simulink model "CarE_Model"  (R2019b)
settings: Solver=VariableStepAuto  StartTime=0.0  StopTime=inf  RelTol=1e-3
(part 1 of 5)
settings Model: EnablePacing=on  Creator=20175127  LastModifiedBy=XPS13
settings DataIOCC: ReturnWorkspaceOutputs=off
settings DebuggingCC: ArithmeticOperatorsInVariantConditions=warning
settings SFSimCC: CustomCodeUndefinedFunction=UseInterfaceOnly

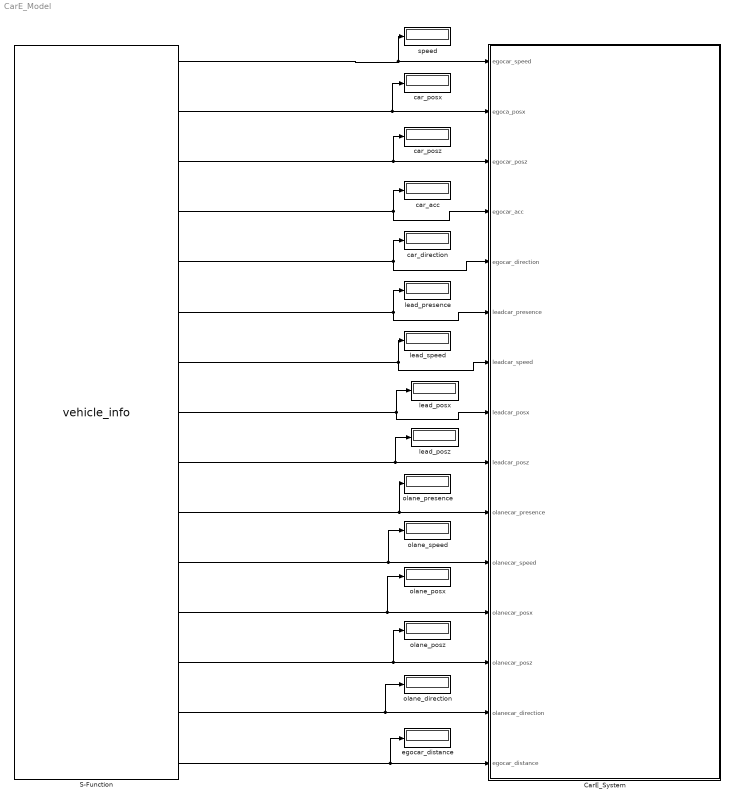
== system CarE_Model ==
  CarE_System : Subsystem
  S-Function : S-Function  FunctionName=vehicle_info  SFunctionDeploymentMode=off  EnableBusSupport=off
  car_acc : Display
  car_direction : Display
  car_posx : Display
  car_posz : Display
  egocar_distance : Display
  lead_posx : Display
  lead_posz : Display
  lead_presence : Display
  lead_speed : Display
      settings: Decimation=5
  olane_direction : Display
  olane_posx : Display
  olane_posz : Display
  olane_presence : Display
  olane_speed : Display
      settings: Decimation=5
  speed : Display
      settings: Decimation=5
  wires:
  S-Function/1 -> CarE_System/1(egocar_speed), speed/1
  S-Function/2 -> car_posx/1, CarE_System/2(egoca_posx)
  S-Function/3 -> CarE_System/3(egocar_posz), car_posz/1
  S-Function/4 -> CarE_System/4(egocar_acc), car_acc/1
  S-Function/5 -> CarE_System/5(egocar_direction), car_direction/1
  S-Function/6 -> CarE_System/6(leadcar_presence), lead_presence/1
  S-Function/7 -> lead_speed/1, CarE_System/7(leadcar_speed)
  S-Function/8 -> CarE_System/8(leadcar_posx), lead_posx/1
  S-Function/9 -> CarE_System/9(leadcar_posz), lead_posz/1
  S-Function/10 -> olane_presence/1, CarE_System/10(olanecar_presence)
  S-Function/11 -> CarE_System/11(olanecar_speed), olane_speed/1
  S-Function/12 -> CarE_System/12(olanecar_posx), olane_posx/1
  S-Function/13 -> olane_posz/1, CarE_System/13(olanecar_posz)
  S-Function/14 -> olane_direction/1, CarE_System/14(olanecar_direction)
  S-Function/15 -> CarE_System/15(egocar_distance), egocar_distance/1

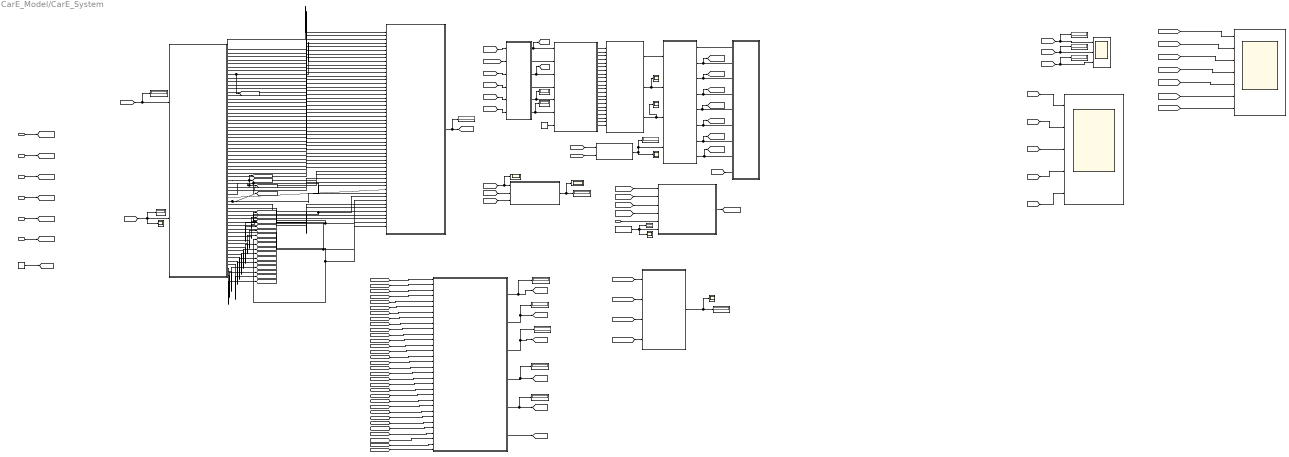
== system CarE_Model/CarE_System ==
  note: Input from unity
  note: output from simulink
  egocar_speed : Inport
  egoca_posx : Inport  Port=2
  egocar_posz : Inport  Port=3
  egocar_acc : Inport  Port=4
  egocar_direction : Inport  Port=5
  leadcar_presence : Inport  Port=6
  leadcar_speed : Inport  Port=7
  leadcar_posx : Inport  Port=8
  leadcar_posz : Inport  Port=9
  olanecar_presence : Inport  Port=10
  olanecar_speed : Inport  Port=11
  olanecar_posx : Inport  Port=12
  olanecar_posz : Inport  Port=13
  olanecar_direction : Inport  Port=14
  egocar_distance : Inport  Port=15
  Display{5..9,11..13} (8 alike) : Display
  Emotion Module : Subsystem
  Emotion_Intensity_Input_Module : Subsystem
  Event_detect_module : Subsystem
  Events-Agent-Event-Action : Scope  NumInputPorts=3
  HF : Display
  HF_normal : Display
  Health_Module_2.0 : Subsystem
  Input_module_2.0 : Subsystem
  MATLAB Function : MATLAB Function  TreatAsAtomicUnit=on
  Mapping Module : Subsystem
  Mood Module : Subsystem
  Optimization_module : Subsystem
  Output Module : Subsystem
  Personality_module : Subsystem
  S-Function1 : S-Function  FunctionName=curve_event  SFunctionDeploymentMode=off  EnableBusSupport=off
  Scope{,1..5} (6 alike) : Scope
  Sress factors : Scope  NumInputPorts=5
  Stress_module : Subsystem
  average_speed_data_mps : Constant  Value=14.72
  basic_emotions : Scope  NumInputPorts=7
  curve_trigger : Display
  fix_LoS : Constant
  gap : Scope
  sf_Env : Display
  sf_VC : Display
  sf_VH : Display
  sf_driving : Display
  sf_total : Display
  speed _CAR : Scope
  utility : Display
  wires:
  Input_module_2.0/16(axle_st) -> Health_Module_2.0/16(axle_st)
  Input_module_2.0/43(bigdata_connection_st) -> Health_Module_2.0/43(bigdata_connection_st), [bigdata_st]
  Input_module_2.0/8(maintanance_periodicity_st) -> Health_Module_2.0/8(maintenance_periodicity_st)
  Input_module_2.0/2(driver_alcohol_st) -> Health_Module_2.0/2(driver_alcohol_st)
  Input_module_2.0/13(service_brak_st) -> Health_Module_2.0/13(serv_brake_PE_st)
  Input_module_2.0/31(telltales_st) -> Health_Module_2.0/31(telltales_st)
  Input_module_2.0/33(wheel_st) -> Health_Module_2.0/33(wheel_st)
  Input_module_2.0/42(software_freq_st) -> Health_Module_2.0/42(software_freq_st)
  Input_module_2.0/51(cab_humiity_st) -> Health_Module_2.0/51(cab_humidity_st)
  Input_module_2.0/14(second_brake_st) -> Health_Module_2.0/14(second_brake_st)
  Input_module_2.0/21(reverse_lamps_st) -> Health_Module_2.0/21(reverse_lamp_st)
  Input_module_2.0/36(chassis_st) -> Health_Module_2.0/36(chassis_st)
  Input_module_2.0/25(steering_st) -> Health_Module_2.0/25(steering_st)
  Input_module_2.0/38(obt_recog_st) -> Health_Module_2.0/38(obt_recog_st)
  Input_module_2.0/32(wheelhub_st) -> Health_Module_2.0/32(wheel_hub_st)
  Input_module_2.0/9(gap_st) -> Health_Module_2.0/9(grap_st), [gap_st]
  Input_module_2.0/24(seat_st) -> Health_Module_2.0/24(seat_st)
  Input_module_2.0/5(driver_workload_st) -> Health_Module_2.0/5(driver_workload_st)
  Input_module_2.0/23(airbag_st) -> Health_Module_2.0/23(airbag_st)
  Input_module_2.0/3(driver_alertness_st) -> Health_Module_2.0/3(driver_alertness_st)
  Input_module_2.0/1(driver_age_st) -> Health_Module_2.0/1(driver_age_st)
  Input_module_2.0/18(door_st) -> Health_Module_2.0/18(door_st)
  Input_module_2.0/41(Friendly_HM_interaction_st) -> Health_Module_2.0/41(friendly_HM_interaction_st)
  Input_module_2.0/4(driver_vision_st) -> Health_Module_2.0/4(driver_vision_st)
  Input_module_2.0/11(vehicle_mass_st) -> Health_Module_2.0/11(vehicle_mass_st)
  Input_module_2.0/39(v2v_st) -> Health_Module_2.0/39(v2v_st), [v2v_st]
  Input_module_2.0/53(weather_st) -> Health_Module_2.0/53(weather_st), [weather_st]
  Input_module_2.0/46(road_surface_st) -> [road_surface_st], Health_Module_2.0/46(road_surface_st)
  Input_module_2.0/48(prob_acc_road_st) -> Health_Module_2.0/48(prob_acc_road_st)
  Input_module_2.0/27(eps_st) -> Health_Module_2.0/27(eps_st)
  Input_module_2.0/49(prob_construction_st) -> Health_Module_2.0/49(prob_construction_st)
  Input_module_2.0/54(time_of_day_st) -> [time_of_day_st], Health_Module_2.0/54(time_of_day_st)
  Input_module_2.0/20(head_lamp_st) -> Health_Module_2.0/20(headlamp_st)
  Input_module_2.0/47(road_condition_st) -> [road_condition_st], Health_Module_2.0/47(road_condition_st)
  Input_module_2.0/40(v2i_st) -> Health_Module_2.0/40(v2i_st), [v2i_st]
  Input_module_2.0/6(driver_emotion_st) -> Health_Module_2.0/6(driver_emotion_st)
  Input_module_2.0/12(brakes_st) -> Health_Module_2.0/12(brakes_st)
  Input_module_2.0/10("speeding_freq_st ") -> Health_Module_2.0/10(speeding_freq_st)
  Input_module_2.0/45(cooperative_driving_st) -> Health_Module_2.0/45(cooperative_driving_st), [cooperative_dr_st]
  Input_module_2.0/7(driver_attitude_st) -> Health_Module_2.0/7(driver_attitude_st)
  Input_module_2.0/19(fog_lamp_st) -> Health_Module_2.0/19(fog_lamp_st)
  Input_module_2.0/44(digital_user_interface_st) -> Health_Module_2.0/44(digital_user_interface_st)
  Input_module_2.0/52(driving_env_contition) -> Health_Module_2.0/52(driving_env_condition_st)
  Input_module_2.0/26(wheel_alignment_st) -> Health_Module_2.0/26(wheel_alignment_st)
  Input_module_2.0/50(cab_temperature_st) -> Health_Module_2.0/50(cab_temperature_st)
  Input_module_2.0/22(belts_st) -> Health_Module_2.0/22(belts_st)
  Input_module_2.0/15(parking_brake_st) -> Health_Module_2.0/15(parkin_brake_st)
  Input_module_2.0/28(streering_wheel_st) -> Health_Module_2.0/28(steering_wheel_st)
  Input_module_2.0/29(stop_lamp_st) -> Health_Module_2.0/29(stop_lamps_st)
  Input_module_2.0/30(suspension_st) -> Health_Module_2.0/30(suspension_st)
  Input_module_2.0/37(noise_st) -> Health_Module_2.0/37(noise_st)
  Input_module_2.0/35(cabine_st) -> Health_Module_2.0/35(cabine_st)
  Input_module_2.0/34(tyre_st) -> Health_Module_2.0/34(tyre_st)
  Input_module_2.0/17(warm_lamp_st) -> Health_Module_2.0/17(warm_lamp_st)
  Emotion Module/21(liking_dec) -> Mood Module/21(liking_dec)
  Emotion Module/8(disappointment_dec) -> Mood Module/8(disappointment_dec)
  Emotion Module/15(admiration_dec) -> Mood Module/15(admiration_dec)
  Mapping Module/8(surprise_val) -> [surprise_val], Output Module/8(surprise_val)
  Mapping Module/5(happiness_val) -> Output Module/5(happiness_val), [happiness_val]
  Emotion Module/11(gloating_dec) -> Mood Module/11(gloating_dec)
  Emotion Module/4(fear_dec) -> Mood Module/4(fear_dec)
  Mapping Module/7(sadness_val) -> Output Module/7(sadness_val), [sadness_val]
  Emotion Module/12(resentment_dec) -> Mood Module/12(resentment_dec)
  Emotion Module/6(fear_confirmed_dec) -> Mood Module/6(fear_confirmed_dec)
  Emotion Module/14(shame_dec) -> Mood Module/14(shame_dec)
  Mapping Module/1(mood_val) -> Output Module/1(mood)
  Mapping Module/6(neutral_val) -> Output Module/6(neutral_val), [neutral_val]
  Mood Module/1(mood) -> Mapping Module/1(mood)
  Emotion Module/20(remorse_dec) -> Mood Module/20(remorse_dec)
  Emotion Module/3(hope_dec) -> Mood Module/3(hope_dec)
  Mood Module/2(contribution) -> Scope1/1, Mapping Module/2(contribution)
  Mood Module/3(index) -> Scope/1, Mapping Module/3(index)
  Emotion Module/7(relief_dec) -> Mood Module/7(relief_dec)
  Emotion Module/18(anger_dec) -> Mood Module/18(anger_dec)
  Emotion Module/19(gratification_dec) -> Mood Module/19(gratification_dec)
  Emotion Module/1(joy_dec) -> Mood Module/1(joy_dec)
  Mapping Module/3(disgust_val) -> Output Module/3(disgust_val), [disgust_val]
  Emotion Module/9(happy_for_dec) -> Mood Module/9(happy_for_dec)
  Emotion Module/5(satisfaction_dec) -> Mood Module/5(satisfaction_dec)
  Emotion Module/2("distress_dec ") -> Mood Module/2(distress_dec)
  Emotion Module/16(reproach_dec) -> Mood Module/16(reproach_dec)
  Emotion Module/13(pride_dec) -> Mood Module/13(pride_dec)
  Mapping Module/2(anger_val) -> [anger_val], Output Module/2(anger_val)
  Mapping Module/4(fear_val) -> [fear_val], Output Module/4(fear_val)
  Emotion Module/22(disliking_dec) -> Mood Module/22(disliking_dec)
  Emotion Module/10(sorry_for_dec) -> Mood Module/10(sorry_for_dec)
  Emotion Module/17(gratitude_dec) -> Mood Module/17(gratitude_dec)
  leadcar_presence/1 -> Event_detect_module/5(leadcar_presence)
  olanecar_presence/1 -> [olanecar_presence]
  S-Function1/1 -> Event_detect_module/6(curve_trigger), curve_trigger/1, Scope4/1
  Health_Module_2.0/1(Health_Factor) -> HF_normal/1, [health_factor]
  egoca_posx/1 -> [egocar_posx]
  egocar_posz/1 -> [egocar_posz]
  egocar_direction/1 -> [egocar_direction]
  egocar_speed/1 -> [egocar_speed]
  Input_module_2.0/55(r_personality) -> [r_personality]
  olanecar_speed/1 -> Stress_module/28(olanecar_speed)
  olanecar_posx/1 -> Stress_module/25(olanecar_posx)
  olanecar_posz/1 -> Stress_module/26(olanecar_posz)
  olanecar_direction/1 -> Stress_module/27(olanecar_direction)
  leadcar_posz/1 -> Stress_module/22(leadcar_posz)
  leadcar_posx/1 -> Stress_module/21(leadcar_posx)
  leadcar_speed/1 -> Stress_module/23(leadcar_speed)
  egocar_acc/1 -> Stress_module/15(egocar_acceleration)
  Event_detect_module/1(event_id) -> [scenario_id]
  Input_module_2.0/56(avg_accident_road) -> [avg_acc_road]
  Input_module_2.0/57(sd_accident_road) -> [sd_acc_road]
  Input_module_2.0/58(accidents_road) -> [acc_road]
  Input_module_2.0/60(Un_Obj_recog) -> [uncertainty_obj_recog]
  Input_module_2.0/59(avg_gap) -> [avg_gap]
  Personality_module/1(Utility) -> Scope2/1, utility/1
  Stress_module/2(Sf_Env) -> [sf_env], sf_Env/1
  Stress_module/1(Sf_VH) -> [sf_vh], sf_VH/1
  Stress_module/5(Sf_driving) -> sf_driving/1, [sf_driving]
  Stress_module/4(sf_VC) -> [sf_vc], sf_VC/1
  Input_module_2.0/64(pedestrian_active) -> [pedestrian_active]
  Input_module_2.0/65(legal_speed) -> [legal_speed]
  Emotion_Intensity_Input_Module/5(LoS) -> Display5/1, Emotion Module/5(LoS)
  Emotion_Intensity_Input_Module/6(LoF) -> Display6/1, Emotion Module/6(LoF)
  Emotion_Intensity_Input_Module/4(action_id) -> Emotion Module/4(action_id)
  Emotion_Intensity_Input_Module/3(event_id) -> [event_id], Emotion Module/3(event_id)
  Emotion_Intensity_Input_Module/2(agent_id) -> Emotion Module/2(agent_id)
  Input_module_2.0/61(rate_acceleration) -> [rate_acceleration]
  Input_module_2.0/62(rate_desceleration) -> [rate_desceleration]
  Input_module_2.0/63(average_speed) -> [avg_speed]
  Stress_module/3(SF_total) -> [stress_factor], sf_total/1
  Input_module_2.0/66(max_car_speed) -> [max_car_speed]
  egocar_distance/1 -> [ego_distance]
  fix_LoS/1 -> Emotion Module/7(fix_loS)
  average_speed_data_mps/1 -> [av_speed_data]
  Optimization_module/1(suggested_speed) -> Scope3/1, Display9/1
  MATLAB Function/1(HF_modified) -> Scope5/1, HF/1, Mapping Module/4(health_factor)
  [ego_distance] -> Input_module_2.0/1(distance), Display8/1
  [ego_distance] -> Stress_module/1(egocar_distance)
  [olanecar_presence] -> Event_detect_module/4(olanecar_presence)
  [olanecar_presence] -> Stress_module/24(olanecar_prescence)
  [egocar_speed] -> speed _CAR/1, Personality_module/1(egocar_speed)
  [egocar_speed] -> Stress_module/9(egocar_speed)
  [egocar_speed] -> Emotion_Intensity_Input_Module/5(egocar_speed)
  [r_personality] -> Personality_module/3(r_personality)
  [max_car_speed] -> Personality_module/2(egocar_max_speed)
  [egocar_posx] -> Event_detect_module/1(egocar_posx)
  [egocar_posx] -> Stress_module/18(egocar_posx)
  [egocar_posz] -> Stress_module/19(egocar_posz)
  [egocar_direction] -> Stress_module/20(egocar_direction)
  [egocar_posz] -> Event_detect_module/2(egocar_posz)
  [egocar_direction] -> Event_detect_module/3(egocar_direction)
  [scenario_id] -> Stress_module/16(event_id)
  [scenario_id] -> Optimization_module/3(event_ID)
  [scenario_id] -> Emotion_Intensity_Input_Module/1(event_ID)
  [scenario_id] -> Events-Agent-Event-Action/1, Display7/1
  Stress_module/6(gap) -> [gap]
  [gap] -> Display11/1, gap/1, Input_module_2.0/2(gap)
  [health_factor] -> MATLAB Function/1(Health_factor)
  [stress_factor] -> Output Module/9(stress_val)
  [stress_factor] -> MATLAB Function/2(SF)
  [stress_factor] -> Emotion_Intensity_Input_Module/3(sf_total)
  [stress_factor] -> Sress factors/5
  [sf_vc] -> Sress factors/3
  [sf_driving] -> Sress factors/4
  [sf_vc] -> Optimization_module/2(SF_VC)
  [sf_vh] -> Optimization_module/1(SF_VH)
  [sf_env] -> Sress factors/2
  [sf_vh] -> Sress factors/1
  [av_speed_data] -> Stress_module/32(avg_speed_data)
  [av_speed_data] -> Optimization_module/4(avgspeed_data)
  [avg_acc_road] -> Stress_module/2(avg_accidents_road)
  [sd_acc_road] -> Stress_module/3(sd_accidents_road)
  [acc_road] -> Stress_module/4(accidents_road)
  [avg_gap] -> Stress_module/17(avg_gap)
  [uncertainty_obj_recog] -> Stress_module/10(un_obj_recog)
  [rate_acceleration] -> Stress_module/30(rate_acceleration)
  [rate_desceleration] -> Stress_module/31(rate_desceleration)
  [avg_speed] -> Stress_module/29(average_speed)
  [pedestrian_active] -> Emotion_Intensity_Input_Module/2(event_0)
  [legal_speed] -> Emotion_Intensity_Input_Module/6(maxlegal_speed)
  [gap_st] -> Emotion_Intensity_Input_Module/4(gap_st)
  [goal_ID] -> Display12/1, Events-Agent-Event-Action/2
  [event_id] -> Events-Agent-Event-Action/3, Display13/1
  Emotion_Intensity_Input_Module/1(goal_id) -> [goal_ID], Emotion Module/1(goal_id)
  [v2v_st] -> Stress_module/11(v2v_st)
  [v2i_st] -> Stress_module/12(v2i_st)
  [bigdata_st] -> Stress_module/13(bigdata_connection_st)
  [cooperative_dr_st] -> Stress_module/14(cooperative_driving_st)
  [road_surface_st] -> Stress_module/5(road_surface_st)
  [road_condition_st] -> Stress_module/6(road_condition_st)
  [weather_st] -> Stress_module/7(weather_condition_st)
  [time_of_day_st] -> Stress_module/8(time_day_st)
  [anger_val] -> basic_emotions/1
  [disgust_val] -> basic_emotions/2
  [fear_val] -> basic_emotions/3
  [happiness_val] -> basic_emotions/4
  [neutral_val] -> basic_emotions/5
  [sadness_val] -> basic_emotions/6
  [surprise_val] -> basic_emotions/7

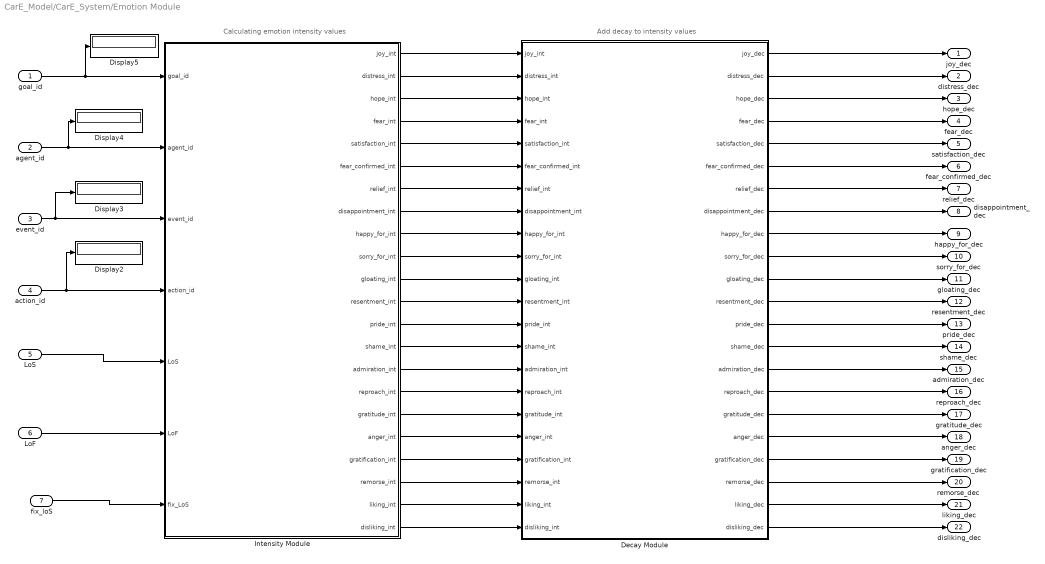
== system CarE_Model/CarE_System/Emotion Module ==
  note: Calculating emotion intensity values
  note: Add decay to intensity values
  goal_id : Inport
  agent_id : Inport  Port=2
  event_id : Inport  Port=3
  action_id : Inport  Port=4
  LoS : Inport  Port=5
  LoF : Inport  Port=6
  fix_loS : Inport  Port=7
  Decay Module : Subsystem
  Display{2..5} (4 alike) : Display
  Intensity Module : Subsystem
  joy_dec : Outport  VectorParamsAs1DForOutWhenUnconnected=off
  "distress_dec " : Outport  Port=2  VectorParamsAs1DForOutWhenUnconnected=off
  hope_dec : Outport  Port=3  VectorParamsAs1DForOutWhenUnconnected=off
  fear_dec : Outport  Port=4  VectorParamsAs1DForOutWhenUnconnected=off
  satisfaction_dec : Outport  Port=5  VectorParamsAs1DForOutWhenUnconnected=off
  fear_confirmed_dec : Outport  Port=6  VectorParamsAs1DForOutWhenUnconnected=off
  relief_dec : Outport  Port=7  VectorParamsAs1DForOutWhenUnconnected=off
  disappointment_dec : Outport  Port=8  VectorParamsAs1DForOutWhenUnconnected=off
  happy_for_dec : Outport  Port=9  VectorParamsAs1DForOutWhenUnconnected=off
  sorry_for_dec : Outport  Port=10  VectorParamsAs1DForOutWhenUnconnected=off
  gloating_dec : Outport  Port=11  VectorParamsAs1DForOutWhenUnconnected=off
  resentment_dec : Outport  Port=12  VectorParamsAs1DForOutWhenUnconnected=off
  pride_dec : Outport  Port=13  VectorParamsAs1DForOutWhenUnconnected=off
  shame_dec : Outport  Port=14  VectorParamsAs1DForOutWhenUnconnected=off
  admiration_dec : Outport  Port=15  VectorParamsAs1DForOutWhenUnconnected=off
  reproach_dec : Outport  Port=16  VectorParamsAs1DForOutWhenUnconnected=off
  gratitude_dec : Outport  Port=17  VectorParamsAs1DForOutWhenUnconnected=off
  anger_dec : Outport  Port=18  VectorParamsAs1DForOutWhenUnconnected=off
  gratification_dec : Outport  Port=19  VectorParamsAs1DForOutWhenUnconnected=off
  remorse_dec : Outport  Port=20  VectorParamsAs1DForOutWhenUnconnected=off
  liking_dec : Outport  Port=21  VectorParamsAs1DForOutWhenUnconnected=off
  disliking_dec : Outport  Port=22  VectorParamsAs1DForOutWhenUnconnected=off
  wires:
  goal_id/1 -> Display5/1, Intensity Module/1(goal_id)
  agent_id/1 -> Intensity Module/2(agent_id), Display4/1
  Intensity Module/1(joy_int) -> Decay Module/1(joy_int)
  Intensity Module/2("distress_int ") -> Decay Module/2(distress_int)
  Intensity Module/3(hope_int) -> Decay Module/3(hope_int)
  Intensity Module/4(fear_int) -> Decay Module/4(fear_int)
  Intensity Module/5(satisfaction_int) -> Decay Module/5(satisfaction_int)
  Intensity Module/6(fear_confirmed_int) -> Decay Module/6(fear_confirmed_int)
  Intensity Module/7(relief_int) -> Decay Module/7(relief_int)
  Intensity Module/8(disappointment_int) -> Decay Module/8(disappointment_int)
  Intensity Module/9(happy_for_int) -> Decay Module/9(happy_for_int)
  Intensity Module/10(sorry_for_int) -> Decay Module/10(sorry_for_int)
  Intensity Module/11(gloating_int) -> Decay Module/11(gloating_int)
  Intensity Module/12(resentment_int) -> Decay Module/12(resentment_int)
  Intensity Module/13(pride_int) -> Decay Module/13(pride_int)
  Intensity Module/14(shame_int) -> Decay Module/14(shame_int)
  Intensity Module/15(admiration_int) -> Decay Module/15(admiration_int)
  Intensity Module/16(reproach_int) -> Decay Module/16(reproach_int)
  Intensity Module/17(gratitude_int) -> Decay Module/17(gratitude_int)
  Intensity Module/18(anger_int) -> Decay Module/18(anger_int)
  Intensity Module/19(gratification_int) -> Decay Module/19(gratification_int)
  Intensity Module/20(remorse_int) -> Decay Module/20(remorse_int)
  Intensity Module/21(liking_int) -> Decay Module/21(liking_int)
  Intensity Module/22(disliking_int) -> Decay Module/22(disliking_int)
  Decay Module/10(sorry_for_dec) -> sorry_for_dec/1
  Decay Module/5(satisfaction_dec) -> satisfaction_dec/1
  Decay Module/11(gloating_dec) -> gloating_dec/1
  Decay Module/7(relief_dec) -> relief_dec/1
  Decay Module/16(reproach_dec) -> reproach_dec/1
  Decay Module/21(liking_dec) -> liking_dec/1
  Decay Module/14(shame_dec) -> shame_dec/1
  Decay Module/13(pride_dec) -> pride_dec/1
  Decay Module/1(joy_dec) -> joy_dec/1
  Decay Module/3(hope_dec) -> hope_dec/1
  Decay Module/17(gratitude_dec) -> gratitude_dec/1
  Decay Module/9(happy_for_dec) -> happy_for_dec/1
  Decay Module/20(remorse_dec) -> remorse_dec/1
  Decay Module/19(gratification_dec) -> gratification_dec/1
  Decay Module/2("distress_dec ") -> "distress_dec "/1
  Decay Module/22(disliking_dec) -> disliking_dec/1
  Decay Module/18(anger_dec) -> anger_dec/1
  Decay Module/6(fear_confirmed_dec) -> fear_confirmed_dec/1
  Decay Module/8(disappointment_dec) -> disappointment_dec/1
  Decay Module/15(admiration_dec) -> admiration_dec/1
  Decay Module/12(resentment_dec) -> resentment_dec/1
  Decay Module/4(fear_dec) -> fear_dec/1
  event_id/1 -> Intensity Module/3(event_id), Display3/1
  action_id/1 -> Intensity Module/4(action_id), Display2/1
  fix_loS/1 -> Intensity Module/7(fix_LoS)
  LoF/1 -> Intensity Module/6(LoF)
  LoS/1 -> Intensity Module/5(LoS)

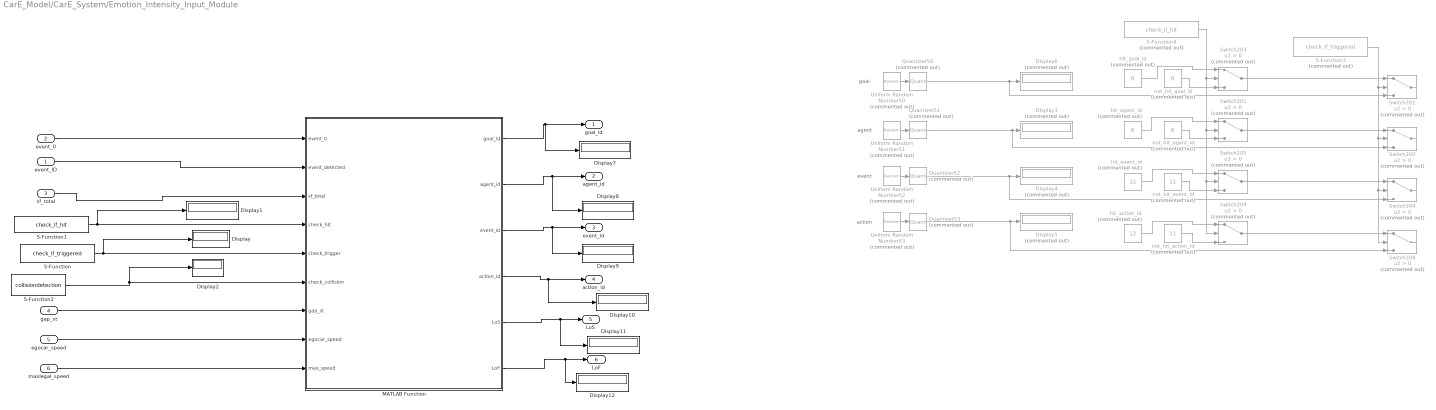
== system CarE_Model/CarE_System/Emotion_Intensity_Input_Module ==
  note: goal
  note: agent
  note: event
  note: action
  event_ID : Inport
  event_0 : Inport  Port=2
  sf_total : Inport  Port=3
  gap_st : Inport  Port=4
  egocar_speed : Inport  Port=5
  maxlegal_speed : Inport  Port=6
  Display{,1..2,7..12} (9 alike) : Display
  Display{3..6} (4 alike) : Display  Commented=on
  MATLAB Function : MATLAB Function  TreatAsAtomicUnit=on
  Quantizer{50..53} (4 alike) : Quantizer  Commented=on  QuantizationInterval=1
  S-Function : S-Function  FunctionName=check_if_triggered  SFunctionDeploymentMode=off  EnableBusSupport=off
  S-Function1 : S-Function  FunctionName=check_if_hit  SFunctionDeploymentMode=off  EnableBusSupport=off
  S-Function2 : S-Function  FunctionName=collisiondetection  SFunctionDeploymentMode=off  EnableBusSupport=off
  S-Function3 : S-Function  Commented=on  FunctionName=check_if_triggered  SFunctionDeploymentMode=off  EnableBusSupport=off
  S-Function4 : S-Function  Commented=on  FunctionName=check_if_hit  SFunctionDeploymentMode=off  EnableBusSupport=off
  Switch{200..205,208..209} (8 alike) : Switch  Commented=on  Criteria=u2 > Threshold
  Uniform Random Number50 : UniformRandomNumber  Commented=on  Minimum=1  Maximum=6  Seed=50  SampleTime=10
  Uniform Random Number51 : UniformRandomNumber  Commented=on  Minimum=1  Maximum=8  Seed=51  SampleTime=10
  Uniform Random Number52 : UniformRandomNumber  Commented=on  Minimum=1  Maximum=12  Seed=52  SampleTime=10
  Uniform Random Number53 : UniformRandomNumber  Commented=on  Minimum=1  Maximum=12  Seed=53  SampleTime=10
  hit_action_id : Constant  Commented=on  Value=12
  hit_agent_id : Constant  Commented=on  Value=6
  hit_event_id : Constant  Commented=on  Value=12
  hit_goal_id : Constant  Commented=on  Value=6
  not_hit_action_id : Constant  Commented=on  Value=11
  not_hit_agent_id : Constant  Commented=on  Value=6
  not_hit_event_id : Constant  Commented=on  Value=11
  not_hit_goal_id : Constant  Commented=on  Value=6
  goal_id : Outport  VectorParamsAs1DForOutWhenUnconnected=off
  agent_id : Outport  Port=2  VectorParamsAs1DForOutWhenUnconnected=off
  event_id : Outport  Port=3  VectorParamsAs1DForOutWhenUnconnected=off
  action_id : Outport  Port=4  VectorParamsAs1DForOutWhenUnconnected=off
  LoS : Outport  Port=5
  LoF : Outport  Port=6
  wires:
  not_hit_event_id/1 -> Switch205/3
  not_hit_action_id/1 -> Switch209/3
  S-Function/1 -> Display/1, MATLAB Function/5(check_trigger)
  hit_agent_id/1 -> Switch201/1
  not_hit_agent_id/1 -> Switch201/3
  Uniform Random Number53/1 -> Quantizer53/1
  Switch209/1 -> Switch208/1
  Switch203/1 -> Switch202/1
  hit_action_id/1 -> Switch209/1
  Switch201/1 -> Switch200/1
  Switch205/1 -> Switch204/1
  Uniform Random Number50/1 -> Quantizer50/1
  hit_goal_id/1 -> Switch203/1
  Uniform Random Number51/1 -> Quantizer51/1
  Quantizer52/1 -> Switch204/3, Display4/1
  S-Function1/1 -> Display1/1, MATLAB Function/4(check_hit)
  Quantizer50/1 -> Switch202/3, Display6/1
  Quantizer53/1 -> Switch208/3, Display5/1
  Uniform Random Number52/1 -> Quantizer52/1
  hit_event_id/1 -> Switch205/1
  Quantizer51/1 -> Switch200/3, Display3/1
  not_hit_goal_id/1 -> Switch203/3
  S-Function2/1 -> MATLAB Function/6(check_collision), Display2/1
  event_ID/1 -> MATLAB Function/2(event_detected)
  maxlegal_speed/1 -> MATLAB Function/9(max_speed)
  egocar_speed/1 -> MATLAB Function/8(egocar_speed)
  gap_st/1 -> MATLAB Function/7(gap_st)
  sf_total/1 -> MATLAB Function/3(sf_total)
  event_0/1 -> MATLAB Function/1(event_0)
  MATLAB Function/6(LoF) -> Display12/1, LoF/1
  MATLAB Function/5(LoS) -> Display11/1, LoS/1
  MATLAB Function/4(action_id) -> Display10/1, action_id/1
  MATLAB Function/3(event_id) -> Display9/1, event_id/1
  MATLAB Function/2(agent_id) -> agent_id/1, Display8/1
  MATLAB Function/1(goal_id) -> Display7/1, goal_id/1
  S-Function3/1 -> Switch208/2, Switch204/2, Switch200/2, Switch202/2
  S-Function4/1 -> Switch209/2, Switch205/2, Switch201/2, Switch203/2

== system CarE_Model/CarE_System/Event_detect_module ==
  egocar_posx : Inport
  egocar_posz : Inport  Port=2
  egocar_direction : Inport  Port=3
  olanecar_presence : Inport  Port=4
  leadcar_presence : Inport  Port=5
  curve_trigger : Inport  Port=6
  MATLAB Function : MATLAB Function  TreatAsAtomicUnit=on
  event_id : Outport
  wires:
  MATLAB Function/1(event_id) -> event_id/1
  curve_trigger/1 -> MATLAB Function/6(turn_trigger)
  leadcar_presence/1 -> MATLAB Function/5(leadcar_presence)
  olanecar_presence/1 -> MATLAB Function/4(olanecar_presence)
  egocar_direction/1 -> MATLAB Function/3(egocar_rot)
  egocar_posz/1 -> MATLAB Function/2(egocar_z)
  egocar_posx/1 -> MATLAB Function/1(egocar_x)

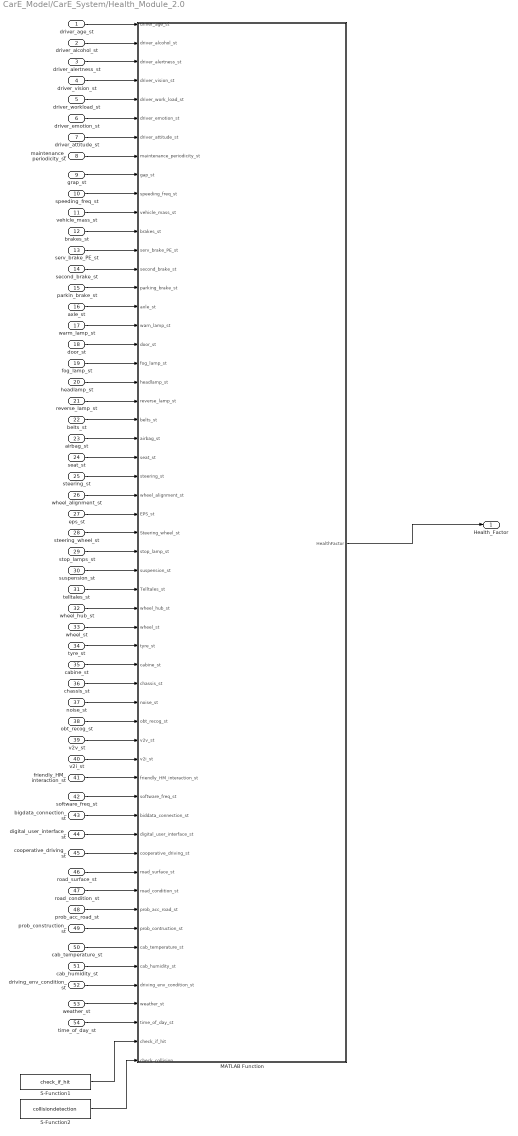
== system CarE_Model/CarE_System/Health_Module_2.0 ==
  driver_age_st : Inport
  driver_alcohol_st : Inport  Port=2
  driver_alertness_st : Inport  Port=3
  driver_vision_st : Inport  Port=4
  driver_workload_st : Inport  Port=5
  driver_emotion_st : Inport  Port=6
  driver_attitude_st : Inport  Port=7
  maintenance_periodicity_st : Inport  Port=8
  grap_st : Inport  Port=9
  speeding_freq_st : Inport  Port=10
  vehicle_mass_st : Inport  Port=11
  brakes_st : Inport  Port=12
  serv_brake_PE_st : Inport  Port=13
  second_brake_st : Inport  Port=14
  parkin_brake_st : Inport  Port=15
  axle_st : Inport  Port=16
  warm_lamp_st : Inport  Port=17
  door_st : Inport  Port=18
  fog_lamp_st : Inport  Port=19
  headlamp_st : Inport  Port=20
  reverse_lamp_st : Inport  Port=21
  belts_st : Inport  Port=22
  airbag_st : Inport  Port=23
  seat_st : Inport  Port=24
  steering_st : Inport  Port=25
  wheel_alignment_st : Inport  Port=26
  eps_st : Inport  Port=27
  steering_wheel_st : Inport  Port=28
  stop_lamps_st : Inport  Port=29
  suspension_st : Inport  Port=30
  telltales_st : Inport  Port=31
  wheel_hub_st : Inport  Port=32
  wheel_st : Inport  Port=33
  tyre_st : Inport  Port=34
  cabine_st : Inport  Port=35
  chassis_st : Inport  Port=36
  noise_st : Inport  Port=37
  obt_recog_st : Inport  Port=38
  v2v_st : Inport  Port=39
  v2i_st : Inport  Port=40
  friendly_HM_interaction_st : Inport  Port=41
  software_freq_st : Inport  Port=42
  bigdata_connection_st : Inport  Port=43
  digital_user_interface_st : Inport  Port=44
  cooperative_driving_st : Inport  Port=45
  road_surface_st : Inport  Port=46
  road_condition_st : Inport  Port=47
  prob_acc_road_st : Inport  Port=48
  prob_construction_st : Inport  Port=49
  cab_temperature_st : Inport  Port=50
  cab_humidity_st : Inport  Port=51
  driving_env_condition_st : Inport  Port=52
  weather_st : Inport  Port=53
  time_of_day_st : Inport  Port=54
  MATLAB Function : MATLAB Function  TreatAsAtomicUnit=on
  S-Function1 : S-Function  FunctionName=check_if_hit  SFunctionDeploymentMode=off  EnableBusSupport=off
  S-Function2 : S-Function  FunctionName=collisiondetection  SFunctionDeploymentMode=off  EnableBusSupport=off
  Health_Factor : Outport
  wires:
  MATLAB Function/1(HealthFactor) -> Health_Factor/1
  time_of_day_st/1 -> MATLAB Function/54(time_of_day_st)
  weather_st/1 -> MATLAB Function/53(weather_st)
  driving_env_condition_st/1 -> MATLAB Function/52(driving_env_condition_st)
  cab_humidity_st/1 -> MATLAB Function/51(cab_humidity_st)
  cab_temperature_st/1 -> MATLAB Function/50(cab_temperature_st)
  prob_construction_st/1 -> MATLAB Function/49(prob_contruction_st)
  prob_acc_road_st/1 -> MATLAB Function/48(prob_acc_road_st)
  road_condition_st/1 -> MATLAB Function/47(road_condition_st)
  road_surface_st/1 -> MATLAB Function/46(road_surface_st)
  cooperative_driving_st/1 -> MATLAB Function/45(cooperative_driving_st)
  digital_user_interface_st/1 -> MATLAB Function/44(digital_user_interface_st)
  bigdata_connection_st/1 -> MATLAB Function/43(biddata_connection_st)
  software_freq_st/1 -> MATLAB Function/42(software_freq_st)
  friendly_HM_interaction_st/1 -> MATLAB Function/41(friendly_HM_interaction_st)
  v2i_st/1 -> MATLAB Function/40(v2i_st)
  v2v_st/1 -> MATLAB Function/39(v2v_st)
  obt_recog_st/1 -> MATLAB Function/38(obt_recog_st)
  noise_st/1 -> MATLAB Function/37(noise_st)
  chassis_st/1 -> MATLAB Function/36(chassis_st)
  cabine_st/1 -> MATLAB Function/35(cabine_st)
  tyre_st/1 -> MATLAB Function/34(tyre_st)
  wheel_st/1 -> MATLAB Function/33(wheel_st)
  wheel_hub_st/1 -> MATLAB Function/32(wheel_hub_st)
  telltales_st/1 -> MATLAB Function/31(Telltales_st)
  suspension_st/1 -> MATLAB Function/30(suspension_st)
  stop_lamps_st/1 -> MATLAB Function/29(stop_lamp_st)
  steering_wheel_st/1 -> MATLAB Function/28(Steering_wheel_st)
  eps_st/1 -> MATLAB Function/27(EPS_st)
  wheel_alignment_st/1 -> MATLAB Function/26(wheel_alignment_st)
  steering_st/1 -> MATLAB Function/25(steering_st)
  seat_st/1 -> MATLAB Function/24(seat_st)
  airbag_st/1 -> MATLAB Function/23(airbag_st)
  belts_st/1 -> MATLAB Function/22(belts_st)
  reverse_lamp_st/1 -> MATLAB Function/21(reverse_lamp_st)
  headlamp_st/1 -> MATLAB Function/20(headlamp_st)
  fog_lamp_st/1 -> MATLAB Function/19(fog_lamp_st)
  door_st/1 -> MATLAB Function/18(door_st)
  warm_lamp_st/1 -> MATLAB Function/17(warn_lamp_st)
  axle_st/1 -> MATLAB Function/16(axle_st)
  parkin_brake_st/1 -> MATLAB Function/15(parking_brake_st)
  second_brake_st/1 -> MATLAB Function/14(second_brake_st)
  serv_brake_PE_st/1 -> MATLAB Function/13(serv_brake_PE_st)
  brakes_st/1 -> MATLAB Function/12(brakes_st)
  vehicle_mass_st/1 -> MATLAB Function/11(vehicle_mass_st)
  speeding_freq_st/1 -> MATLAB Function/10(speeding_freq_st)
  grap_st/1 -> MATLAB Function/9(gap_st)
  maintenance_periodicity_st/1 -> MATLAB Function/8(maintenance_periodicity_st)
  driver_attitude_st/1 -> MATLAB Function/7(driver_attitude_st)
  driver_emotion_st/1 -> MATLAB Function/6(driver_emotion_st)
  driver_workload_st/1 -> MATLAB Function/5(driver_work_load_st)
  driver_vision_st/1 -> MATLAB Function/4(driver_vision_st)
  driver_alertness_st/1 -> MATLAB Function/3(driver_alertness_st)
  driver_alcohol_st/1 -> MATLAB Function/2(driver_alcohol_st)
  driver_age_st/1 -> MATLAB Function/1(driver_age_st)
  S-Function1/1 -> MATLAB Function/55(check_if_hit)
  S-Function2/1 -> MATLAB Function/56(check_collision)

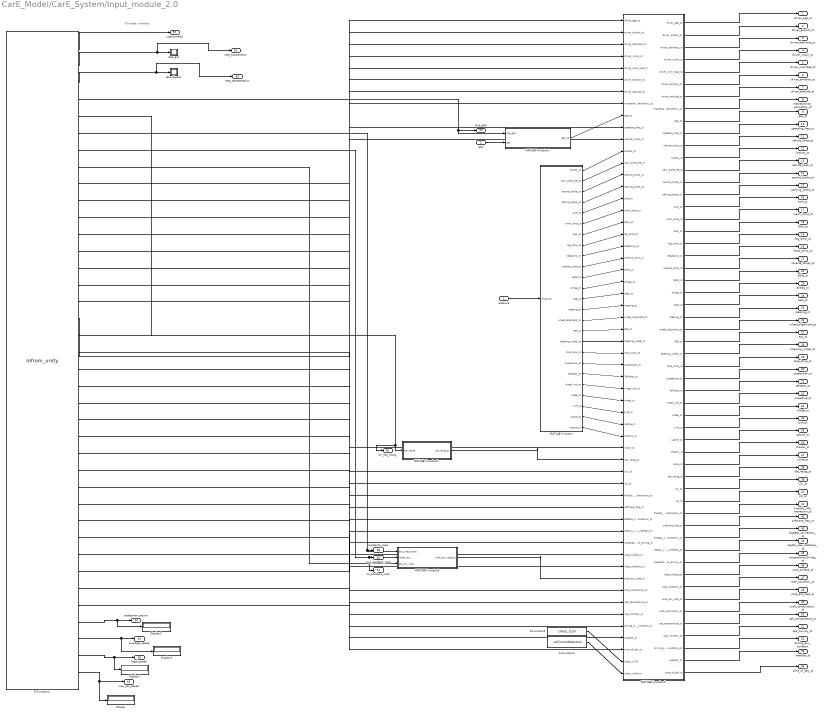
== system CarE_Model/CarE_System/Input_module_2.0 ==
  note: NO-state variables
  distance : Inport
  gap : Inport  Port=2
  Display{,1..3} (4 alike) : Display
  MATLAB Function : MATLAB Function  TreatAsAtomicUnit=on
  MATLAB Function1 : MATLAB Function  TreatAsAtomicUnit=on
  MATLAB Function2 : MATLAB Function  TreatAsAtomicUnit=on
  MATLAB Function3 : MATLAB Function  TreatAsAtomicUnit=on
  MATLAB Function4 : MATLAB Function  TreatAsAtomicUnit=on
  S-Function1 : S-Function  FunctionName=infrom_unity  SFunctionDeploymentMode=off  EnableBusSupport=off
  S-Function2 : S-Function  FunctionName=check_if_hit  SFunctionDeploymentMode=off  EnableBusSupport=off
  S-Function3 : S-Function  FunctionName=collisiondetection  SFunctionDeploymentMode=off  EnableBusSupport=off
  rate_acc : Display
  rate_desacc : Display
  driver_age_st : Outport
  driver_alcohol_st : Outport  Port=2
  driver_alertness_st : Outport  Port=3
  driver_vision_st : Outport  Port=4
  driver_workload_st : Outport  Port=5
  driver_emotion_st : Outport  Port=6
  driver_attitude_st : Outport  Port=7
  maintanance_periodicity_st : Outport  Port=8
  gap_st : Outport  Port=9
  "speeding_freq_st " : Outport  Port=10
  vehicle_mass_st : Outport  Port=11
  brakes_st : Outport  Port=12
  service_brak_st : Outport  Port=13
  second_brake_st : Outport  Port=14
  parking_brake_st : Outport  Port=15
  axle_st : Outport  Port=16
  warm_lamp_st : Outport  Port=17
  door_st : Outport  Port=18
  fog_lamp_st : Outport  Port=19
  head_lamp_st : Outport  Port=20
  reverse_lamps_st : Outport  Port=21
  belts_st : Outport  Port=22
  airbag_st : Outport  Port=23
  seat_st : Outport  Port=24
  steering_st : Outport  Port=25
  wheel_alignment_st : Outport  Port=26
  eps_st : Outport  Port=27
  streering_wheel_st : Outport  Port=28
  stop_lamp_st : Outport  Port=29
  suspension_st : Outport  Port=30
  telltales_st : Outport  Port=31
  wheelhub_st : Outport  Port=32
  wheel_st : Outport  Port=33
  tyre_st : Outport  Port=34
  cabine_st : Outport  Port=35
  chassis_st : Outport  Port=36
  noise_st : Outport  Port=37
  obt_recog_st : Outport  Port=38
  v2v_st : Outport  Port=39
  v2i_st : Outport  Port=40
  Friendly_HM_interaction_st : Outport  Port=41
  software_freq_st : Outport  Port=42
  bigdata_connection_st : Outport  Port=43
  digital_user_interface_st : Outport  Port=44
  cooperative_driving_st : Outport  Port=45
  road_surface_st : Outport  Port=46
  road_condition_st : Outport  Port=47
  prob_acc_road_st : Outport  Port=48
  prob_construction_st : Outport  Port=49
  cab_temperature_st : Outport  Port=50
  cab_humiity_st : Outport  Port=51
  driving_env_contition : Outport  Port=52
  weather_st : Outport  Port=53
  time_of_day_st : Outport  Port=54
  r_personality : Outport  Port=55
  avg_accident_road : Outport  Port=56
  sd_accident_road : Outport  Port=57
  accidents_road : Outport  Port=58
  avg_gap : Outport  Port=59
  Un_Obj_recog : Outport  Port=60
  rate_acceleration : Outport  Port=61
  rate_desceleration : Outport  Port=62
  average_speed : Outport  Port=63
  pedestrian_active : Outport  Port=64
  legal_speed : Outport  Port=65
  max_car_speed : Outport  Port=66
  wires:
  S-Function1/6 -> accidents_road/1, MATLAB Function3/1(acc_road_today)
  S-Function1/2 -> rate_acceleration/1, rate_acc/1
  S-Function1/7 -> MATLAB Function3/2(mean_acc), avg_accident_road/1
  S-Function1/3 -> rate_desceleration/1, rate_desacc/1
  S-Function1/8 -> MATLAB Function3/3(SD_acc_road), sd_accident_road/1
  S-Function1/4 -> MATLAB Function1/1(avg_gap), avg_gap/1
  S-Function1/1 -> r_personality/1
  S-Function1/9 -> MATLAB Function4/1("driver_age_st ")
  distance/1 -> MATLAB Function/1(distance)
  MATLAB Function/1(brakes_st) -> MATLAB Function4/12("brakes_st ")
  MATLAB Function/2(serv_brake_PE_st) -> MATLAB Function4/13("serv_brake_PE_st ")
  MATLAB Function/3(second_brake_st) -> MATLAB Function4/14("second_brake_st ")
  MATLAB Function/4(parking_brake_st) -> MATLAB Function4/15("parking_brake_st ")
  MATLAB Function/5(axle_st) -> MATLAB Function4/16("axle_st ")
  MATLAB Function/6(warn_lamp_st) -> MATLAB Function4/17("warn_lamp_st ")
  MATLAB Function/7(door_st) -> MATLAB Function4/18("door_st ")
  MATLAB Function/8(fog_lamp_st) -> MATLAB Function4/19("fog_lamp_st ")
  MATLAB Function/9(headlamp_st) -> MATLAB Function4/20("headlamp_st ")
  gap/1 -> MATLAB Function1/2(gap)
  MATLAB Function1/1(gap_st) -> MATLAB Function4/9("gap_st ")
  S-Function1/10 -> MATLAB Function4/6("driver_emotion_st ")
  S-Function1/11 -> MATLAB Function4/2("driver_alcohol_st ")
  S-Function1/12 -> MATLAB Function4/3("driver_alertness_st ")
  S-Function1/13 -> MATLAB Function4/4("driver_vision_st ")
  S-Function1/14 -> MATLAB Function4/5("driver_work_load_st ")
  S-Function1/15 -> MATLAB Function4/7("driver_attitude_st ")
  S-Function1/16 -> MATLAB Function4/8("maintenance_periodicity_st ")
  S-Function1/17 -> MATLAB Function4/10("speeding_freq_st ")
  S-Function1/18 -> MATLAB Function4/11("vehicle_mass_st ")
  MATLAB Function/10(reverse_lamp_st) -> MATLAB Function4/21("reverse_lamp_st ")
  MATLAB Function/11(belts_st) -> MATLAB Function4/22("belts_st ")
  MATLAB Function/12(airbag_st) -> MATLAB Function4/23("airbag_st ")
  MATLAB Function/13(seat_st) -> MATLAB Function4/24("seat_st ")
  MATLAB Function/14(steering_st) -> MATLAB Function4/25("steering_st ")
  MATLAB Function/15(wheel_alignment_st) -> MATLAB Function4/26("wheel_alignment_st ")
  MATLAB Function/16(EPS_st) -> MATLAB Function4/27("EPS_st ")
  MATLAB Function/17(Steering_wheel_st) -> MATLAB Function4/28("Steering_wheel_st ")
  MATLAB Function/18(stop_lamp_st) -> MATLAB Function4/29("stop_lamp_st ")
  MATLAB Function/19(suspension_st) -> MATLAB Function4/30("suspension_st ")
  MATLAB Function/20(Telltales_st) -> MATLAB Function4/31("Telltales_st ")
  MATLAB Function/21(wheel_hub_st) -> MATLAB Function4/32("wheel_hub_st ")
  MATLAB Function/22(wheel_st) -> MATLAB Function4/33("wheel_st ")
  MATLAB Function/23(tyre_st) -> MATLAB Function4/34("tyre_st ")
  MATLAB Function/24(cabine_st) -> MATLAB Function4/35("cabine_st ")
  MATLAB Function/25(chassis_st) -> MATLAB Function4/36("chassis_st ")
  S-Function1/19 -> MATLAB Function4/37("noise_st ")
  MATLAB Function2/1(ob_recog_st) -> MATLAB Function4/38("obt_recog_st ")
  S-Function1/5 -> MATLAB Function2/1(obt_recog), Un_Obj_recog/1
  S-Function1/23 -> MATLAB Function4/39("v2v_st ")
  S-Function1/24 -> MATLAB Function4/40("v2i_st ")
  S-Function1/20 -> MATLAB Function4/41("friendly_HM_interaction_st ")
  S-Function1/21 -> MATLAB Function4/42("software_freq_st ")
  S-Function1/25 -> MATLAB Function4/43("biddata_connection_st ")
  S-Function1/22 -> MATLAB Function4/44("digital_user_interface_st ")
  S-Function1/26 -> MATLAB Function4/45("cooperative_driving_st ")
  MATLAB Function3/1(prob_acc_road_st) -> MATLAB Function4/48("prob_acc_road_st ")
  S-Function1/27 -> MATLAB Function4/49("prob_contruction_st ")
  S-Function1/28 -> MATLAB Function4/50("cab_temperature_st ")
  S-Function1/29 -> MATLAB Function4/51("cab_humidity_st ")
  S-Function1/30 -> MATLAB Function4/52("driving_env_condition_st ")
  S-Function1/31 -> MATLAB Function4/46("road_surface_st ")
  S-Function1/32 -> MATLAB Function4/47("road_condition_st ")
  S-Function1/33 -> MATLAB Function4/53("weather_st ")
  S-Function1/34 -> MATLAB Function4/54("time_of_day_st ")
  S-Function2/1 -> MATLAB Function4/55(check_if_hit)
  S-Function3/1 -> MATLAB Function4/56(check_collision)
  MATLAB Function4/1(driver_age_st) -> driver_age_st/1
  MATLAB Function4/2(driver_alcohol_st) -> driver_alcohol_st/1
  MATLAB Function4/3(driver_alertness_st) -> driver_alertness_st/1
  MATLAB Function4/4(driver_vision_st) -> driver_vision_st/1
  MATLAB Function4/5(driver_work_load_st) -> driver_workload_st/1
  MATLAB Function4/6(driver_emotion_st) -> driver_emotion_st/1
  MATLAB Function4/7(driver_attitude_st) -> driver_attitude_st/1
  MATLAB Function4/8(maintenance_periodicity_st) -> maintanance_periodicity_st/1
  MATLAB Function4/12(brakes_st) -> brakes_st/1
  MATLAB Function4/13(serv_brake_PE_st) -> service_brak_st/1
  MATLAB Function4/14(second_brake_st) -> second_brake_st/1
  MATLAB Function4/15(parking_brake_st) -> parking_brake_st/1
  MATLAB Function4/16(axle_st) -> axle_st/1
  MATLAB Function4/17(warn_lamp_st) -> warm_lamp_st/1
  MATLAB Function4/19(fog_lamp_st) -> fog_lamp_st/1
  MATLAB Function4/18(door_st) -> door_st/1
  MATLAB Function4/20(headlamp_st) -> head_lamp_st/1
  MATLAB Function4/21(reverse_lamp_st) -> reverse_lamps_st/1
  MATLAB Function4/22(belts_st) -> belts_st/1
  MATLAB Function4/23(airbag_st) -> airbag_st/1
  MATLAB Function4/24(seat_st) -> seat_st/1
  MATLAB Function4/25(steering_st) -> steering_st/1
  MATLAB Function4/26(wheel_alignment_st) -> wheel_alignment_st/1
  MATLAB Function4/27(EPS_st) -> eps_st/1
  MATLAB Function4/28(Steering_wheel_st) -> streering_wheel_st/1
  MATLAB Function4/29(stop_lamp_st) -> stop_lamp_st/1
  MATLAB Function4/30(suspension_st) -> suspension_st/1
  MATLAB Function4/31(Telltales_st) -> telltales_st/1
  MATLAB Function4/32(wheel_hub_st) -> wheelhub_st/1
  MATLAB Function4/33(wheel_st) -> wheel_st/1
  MATLAB Function4/34(tyre_st) -> tyre_st/1
  MATLAB Function4/35(cabine_st) -> cabine_st/1
  MATLAB Function4/36(chassis_st) -> chassis_st/1
  MATLAB Function4/9(gap_st) -> gap_st/1
  MATLAB Function4/10(speeding_freq_st) -> "speeding_freq_st "/1
  MATLAB Function4/11(vehicle_mass_st) -> vehicle_mass_st/1
  MATLAB Function4/37(noise_st) -> noise_st/1
  MATLAB Function4/38(obt_recog_st) -> obt_recog_st/1
  MATLAB Function4/39(v2v_st) -> v2v_st/1
  MATLAB Function4/40(v2i_st) -> v2i_st/1
  MATLAB Function4/41(friendly_HM_interaction_st) -> Friendly_HM_interaction_st/1
  MATLAB Function4/42(software_freq_st) -> software_freq_st/1
  MATLAB Function4/43(biddata_connection_st) -> bigdata_connection_st/1
  MATLAB Function4/44(digital_user_interface_st) -> digital_user_interface_st/1
  MATLAB Function4/45(cooperative_driving_st) -> cooperative_driving_st/1
  MATLAB Function4/47(road_condition_st) -> road_condition_st/1
  MATLAB Function4/46(road_surface_st) -> road_surface_st/1
  MATLAB Function4/48(prob_acc_road_st) -> prob_acc_road_st/1
  MATLAB Function4/49(prob_contruction_st) -> prob_construction_st/1
  MATLAB Function4/50(cab_temperature_st) -> cab_temperature_st/1
  MATLAB Function4/51(cab_humidity_st) -> cab_humiity_st/1
  MATLAB Function4/52(driving_env_condition_st) -> driving_env_contition/1
  MATLAB Function4/53(weather_st) -> weather_st/1
  MATLAB Function4/54(time_of_day_st) -> time_of_day_st/1
  S-Function1/36 -> Display2/1, average_speed/1
  S-Function1/38 -> max_car_speed/1, Display/1
  S-Function1/37 -> Display1/1, legal_speed/1
  S-Function1/35 -> Display3/1, pedestrian_active/1

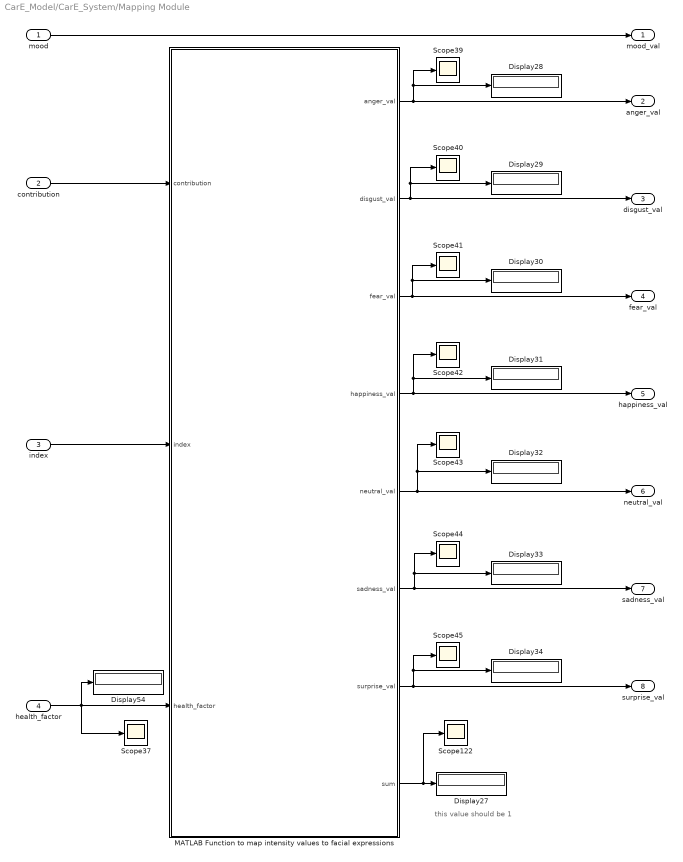
== system CarE_Model/CarE_System/Mapping Module ==
  note: this value should be 1
  mood : Inport
  contribution : Inport  Port=2
  index : Inport  Port=3
  health_factor : Inport  Port=4
  Display{27..34,54} (9 alike) : Display
  MATLAB Function to map intensity values to facial expressions : MATLAB Function  TreatAsAtomicUnit=on
  Scope{37,39..45,122} (9 alike) : Scope
  mood_val : Outport  VectorParamsAs1DForOutWhenUnconnected=off
  anger_val : Outport  Port=2  VectorParamsAs1DForOutWhenUnconnected=off
  disgust_val : Outport  Port=3  VectorParamsAs1DForOutWhenUnconnected=off
  fear_val : Outport  Port=4  VectorParamsAs1DForOutWhenUnconnected=off
  happiness_val : Outport  Port=5  VectorParamsAs1DForOutWhenUnconnected=off
  neutral_val : Outport  Port=6  VectorParamsAs1DForOutWhenUnconnected=off
  sadness_val : Outport  Port=7  VectorParamsAs1DForOutWhenUnconnected=off
  surprise_val : Outport  Port=8  VectorParamsAs1DForOutWhenUnconnected=off
  wires:
  MATLAB Function to map intensity values to facial expressions/5(neutral_val) -> neutral_val/1, Scope43/1, Display32/1
  MATLAB Function to map intensity values to facial expressions/4(happiness_val) -> happiness_val/1, Display31/1, Scope42/1
  MATLAB Function to map intensity values to facial expressions/2(disgust_val) -> disgust_val/1, Display29/1, Scope40/1
  MATLAB Function to map intensity values to facial expressions/6(sadness_val) -> sadness_val/1, Scope44/1, Display33/1
  MATLAB Function to map intensity values to facial expressions/8(sum) -> Scope122/1, Display27/1
  contribution/1 -> MATLAB Function to map intensity values to facial expressions/1(contribution)
  health_factor/1 -> Display54/1, MATLAB Function to map intensity values to facial expressions/3(health_factor), Scope37/1
  index/1 -> MATLAB Function to map intensity values to facial expressions/2(index)
  MATLAB Function to map intensity values to facial expressions/7(surprise_val) -> surprise_val/1, Display34/1, Scope45/1
  MATLAB Function to map intensity values to facial expressions/3(fear_val) -> fear_val/1, Display30/1, Scope41/1
  MATLAB Function to map intensity values to facial expressions/1(anger_val) -> anger_val/1, Scope39/1, Display28/1
  mood/1 -> mood_val/1

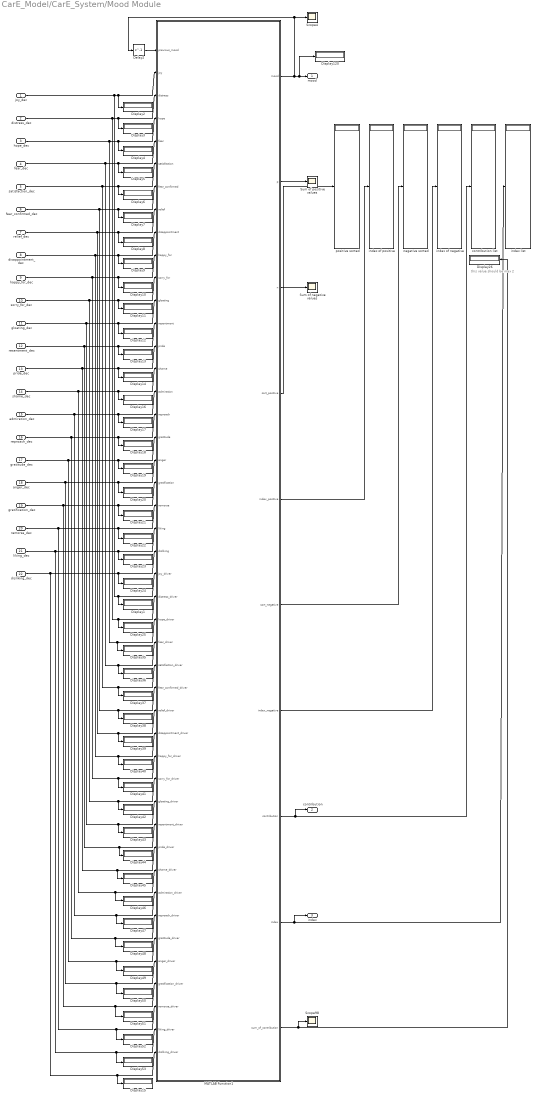
== system CarE_Model/CarE_System/Mood Module ==
  note: this value should be max 2
  joy_dec : Inport
  distress_dec : Inport  Port=2
  hope_dec : Inport  Port=3
  fear_dec : Inport  Port=4
  satisfaction_dec : Inport  Port=5
  fear_confirmed_dec : Inport  Port=6
  relief_dec : Inport  Port=7
  disappointment_dec : Inport  Port=8
  happy_for_dec : Inport  Port=9
  sorry_for_dec : Inport  Port=10
  gloating_dec : Inport  Port=11
  resentment_dec : Inport  Port=12
  pride_dec : Inport  Port=13
  shame_dec : Inport  Port=14
  admiration_dec : Inport  Port=15
  reproach_dec : Inport  Port=16
  gratitude_dec : Inport  Port=17
  anger_dec : Inport  Port=18
  gratification_dec : Inport  Port=19
  remorse_dec : Inport  Port=20
  liking_dec : Inport  Port=21
  disliking_dec : Inport  Port=22
  Delay2 : Delay  DelayLength=1  InitialCondition=0
  Display{1..26,35..53,120} (46 alike) : Display
  MATLAB Function1 : MATLAB Function  TreatAsAtomicUnit=on
  Scope4 : Scope
  Scope98 : Scope
  Sum of negative values : Scope
  Sum of positive values : Scope
  contribution list : Display
  index list : Display
  index of negative : Display
  index of positive : Display
  negative sorted : Display
  positive sorted : Display
  mood : Outport  VectorParamsAs1DForOutWhenUnconnected=off
  contribution : Outport  Port=2  VectorParamsAs1DForOutWhenUnconnected=off
  index : Outport  Port=3  VectorParamsAs1DForOutWhenUnconnected=off
  wires:
  shame_dec/1 -> Display46/1, MATLAB Function1/37(shame_driver), Display16/1, MATLAB Function1/15(shame)
  relief_dec/1 -> Display39/1, MATLAB Function1/30(relief_driver), Display8/1, MATLAB Function1/8(relief)
  MATLAB Function1/2(p) -> Sum of positive values/1
  MATLAB Function1/3(n) -> Sum of negative values/1
  sorry_for_dec/1 -> Display42/1, MATLAB Function1/33(sorry_for_driver), Display11/1, MATLAB Function1/11(sorry_for)
  anger_dec/1 -> Display50/1, MATLAB Function1/41(anger_driver), Display20/1, MATLAB Function1/19(anger)
  distress_dec/1 -> MATLAB Function1/25(distress_driver), Display25/1, Display3/1, MATLAB Function1/3(distress)
  fear_confirmed_dec/1 -> Display38/1, MATLAB Function1/29(fear_confirmed_driver), Display7/1, MATLAB Function1/7(fear_confirmed)
  MATLAB Function1/7(index_negative) -> index of negative/1
  MATLAB Function1/8(contribution) -> contribution/1, contribution list/1
  MATLAB Function1/5(index_positive) -> index of positive/1
  remorse_dec/1 -> Display52/1, MATLAB Function1/43(remorse_driver), Display22/1, MATLAB Function1/21(remorse)
  MATLAB Function1/4(sort_positive) -> positive sorted/1
  satisfaction_dec/1 -> Display37/1, MATLAB Function1/28(satisfaction_driver), Display6/1, MATLAB Function1/6(satisfaction)
  disappointment_dec/1 -> MATLAB Function1/9(disappointment), Display9/1, Display40/1, MATLAB Function1/31(disappointment_driver)
  liking_dec/1 -> Display53/1, MATLAB Function1/44(liking_driver), Display23/1, MATLAB Function1/22(liking)
  disliking_dec/1 -> Display15/1, MATLAB Function1/45(disliking_driver), Display24/1, MATLAB Function1/23(disliking)
  admiration_dec/1 -> Display17/1, MATLAB Function1/16(admiration), Display47/1, MATLAB Function1/38(admiration_driver)
  gratitude_dec/1 -> MATLAB Function1/40(gratitude_driver), Display49/1, MATLAB Function1/18(gratitude), Display19/1
  resentment_dec/1 -> Display13/1, MATLAB Function1/13(resentment), Display44/1, MATLAB Function1/35(resentment_driver)
  MATLAB Function1/6(sort_negative) -> negative sorted/1
  gratification_dec/1 -> Display51/1, MATLAB Function1/42(gratification_driver), Display21/1, MATLAB Function1/20(gratification)
  pride_dec/1 -> Display45/1, MATLAB Function1/36(pride_driver), Display14/1, MATLAB Function1/14(pride)
  Delay2/1 -> MATLAB Function1/1(previous_mood)
  MATLAB Function1/1(mood) -> mood/1, Display120/1, Delay2/1, Scope4/1
  hope_dec/1 -> Display35/1, MATLAB Function1/26(hope_driver), Display4/1, MATLAB Function1/4(hope)
  happy_for_dec/1 -> MATLAB Function1/32(happy_for_driver), Display41/1, Display10/1, MATLAB Function1/10(happy_for)
  MATLAB Function1/9(index) -> index/1, index list/1
  MATLAB Function1/10(sum_of_contribution) -> Scope98/1, Display26/1
  fear_dec/1 -> Display36/1, MATLAB Function1/27(fear_driver), Display5/1, MATLAB Function1/5(fear)
  gloating_dec/1 -> Display43/1, MATLAB Function1/34(gloating_driver), Display12/1, MATLAB Function1/12(gloating)
  reproach_dec/1 -> Display18/1, MATLAB Function1/17(reproach), Display48/1, MATLAB Function1/39(reproach_driver)
  joy_dec/1 -> Display1/1, MATLAB Function1/24(joy_driver), Display2/1, MATLAB Function1/2(joy)
